simulink model "Cmd_HacheurF"  (R2016a)
settings: Solver=ode1  StartTime=0.0  StopTime=0.05  FixedStep=Te  RelTol=1e-3
values from neighbouring files (symbols this model uses):
  A = [-R/L -1/L;1/Cdc -1/(Cdc*Rch)]    [Param.m]
  Ad = [1-Te*R/L -Te/L;Te/Cdc 1-Te/(Cdc*Rch)]    [Param.m]
  B = [1/L;0]    [Param.m]
  Bd = [Te/L;0]    [Param.m]
  C = [0 1]    [Param.m]
  Cd = [0 1]    [Param.m]
  Cdc = 200e-6    (= 0.0002)    [Param.m]
  K = place(A,B,[p1BF;p2BF])    [Param.m]
  L = 12.5e-3    (= 0.0125)    [Param.m]
  LOBS = LOBS_T'    [Param.m]
  LOBSd = Te*LOBS    [Param.m]
  N = inv(-C*inv(A-B*K)*B)    [Param.m]
  R = 0.3    [Param.m]
  Rch = 50    [Param.m]
  Te = 20e-6    (= 2e-05)    [Param.m]
  X_0 = [0;0]    [Param.m]
settings Model: Creator=Wissem  LastModifiedBy=dell

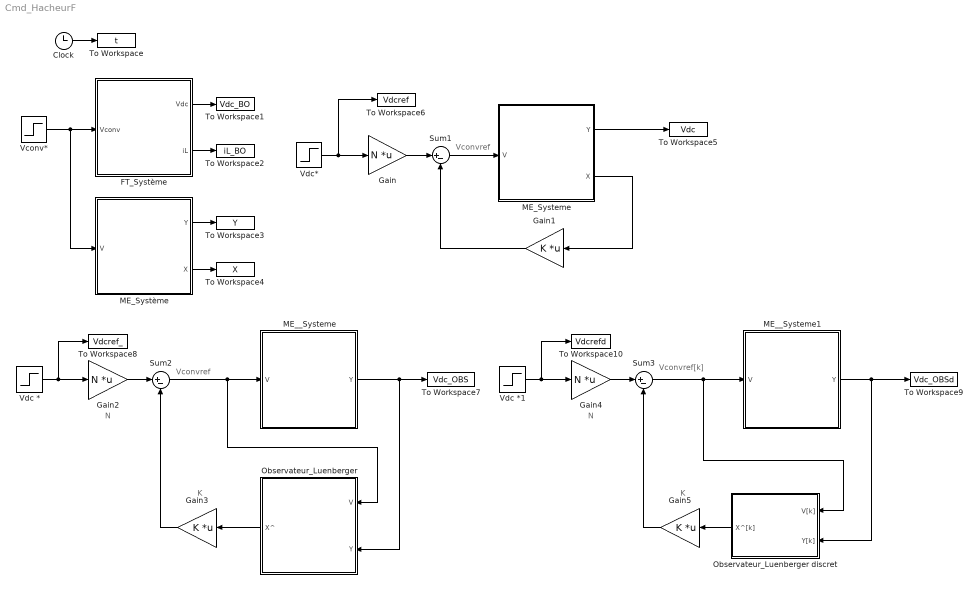
== system Cmd_HacheurF ==
  note: N
  note: K
  note: Vconvref
  note: Vconvref
  note: N
  note: K
  note: Vconvref[k]
  Clock : Clock
  FT_Système : Subsystem
  Gain : Gain  Gain=N  Multiplication=Matrix(K*u)
  Gain1 : Gain  Gain=K  Multiplication=Matrix(K*u) (u vector)
  Gain2 : Gain  Gain=N  Multiplication=Matrix(K*u)
  Gain3 : Gain  Gain=K  Multiplication=Matrix(K*u) (u vector)
  Gain4 : Gain  Gain=N  Multiplication=Matrix(K*u)
  Gain5 : Gain  Gain=K  Multiplication=Matrix(K*u) (u vector)
  ME_Systeme : Subsystem
  ME_Système : Subsystem
  ME__Systeme : Subsystem
  ME__Systeme1 : Subsystem
  Observateur_Luenberger : Subsystem
  Observateur_Luenberger discret : Subsystem
  Sum1 : Sum  Inputs=|+-
  Sum2 : Sum  Inputs=|+-
  Sum3 : Sum  Inputs=|+-
  To Workspace : ToWorkspace  VariableName=t  SampleTime=-1
  To Workspace1 : ToWorkspace  VariableName=Vdc_BO  SampleTime=-1
  To Workspace10 : ToWorkspace  VariableName=Vdcrefd  SampleTime=-1
  To Workspace2 : ToWorkspace  VariableName=iL_BO  SampleTime=-1
  To Workspace3 : ToWorkspace  VariableName=Y  SampleTime=-1
  To Workspace4 : ToWorkspace  VariableName=X  SampleTime=-1
  To Workspace5 : ToWorkspace  VariableName=Vdc  SampleTime=-1
  To Workspace6 : ToWorkspace  VariableName=Vdcref  SampleTime=-1
  To Workspace7 : ToWorkspace  VariableName=Vdc_OBS  SampleTime=-1
  To Workspace8 : ToWorkspace  VariableName=Vdcref_  SampleTime=-1
  To Workspace9 : ToWorkspace  VariableName=Vdc_OBSd  SampleTime=-1
  Vconv* : Step  Time=0  After=100  SampleTime=0
  Vdc * : Step  Time=0  After=100  SampleTime=0
  Vdc *1 : Step  Time=0  After=100  SampleTime=0
  Vdc* : Step  Time=0  After=100  SampleTime=0
  wires:
  Vconv*/1 -> ME_Système/1(V), FT_Système/1(Vconv)
  Clock/1 -> To Workspace/1
  FT_Système/1(Vdc) -> To Workspace1/1
  FT_Système/2(iL) -> To Workspace2/1
  ME_Système/1(Y) -> To Workspace3/1
  ME_Système/2(X) -> To Workspace4/1
  Gain1/1 -> Sum1/2
  Gain/1 -> Sum1/1
  Vdc*/1 -> To Workspace6/1, Gain/1
  Sum1/1 -> ME_Systeme/1(V)
  ME_Systeme/1(Y) -> To Workspace5/1
  ME_Systeme/2(X) -> Gain1/1
  Gain3/1 -> Sum2/2
  Gain2/1 -> Sum2/1
  Vdc */1 -> Gain2/1, To Workspace8/1
  Sum2/1 -> Observateur_Luenberger/1(V), ME__Systeme/1(V)
  ME__Systeme/1(Y) -> Observateur_Luenberger/2(Y), To Workspace7/1
  Observateur_Luenberger/1(X^) -> Gain3/1
  Gain5/1 -> Sum3/2
  Gain4/1 -> Sum3/1
  Vdc *1/1 -> To Workspace10/1, Gain4/1
  Sum3/1 -> Observateur_Luenberger discret/1(V[k]), ME__Systeme1/1(V)
  ME__Systeme1/1(Y) -> Observateur_Luenberger discret/2(Y[k]), To Workspace9/1
  Observateur_Luenberger discret/1(X^[k]) -> Gain5/1

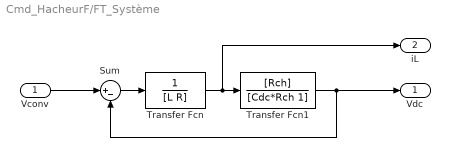
== system Cmd_HacheurF/FT_Système ==
  Vconv : Inport
  Sum : Sum  Inputs=|+-
  Transfer Fcn : TransferFcn  Denominator=[L R]
  Transfer Fcn1 : TransferFcn  Numerator=[Rch]  Denominator=[Cdc*Rch 1]
  Vdc : Outport
  iL : Outport  Port=2
  wires:
  Transfer Fcn/1 -> iL/1, Transfer Fcn1/1
  Transfer Fcn1/1 -> Vdc/1, Sum/2
  Sum/1 -> Transfer Fcn/1
  Vconv/1 -> Sum/1

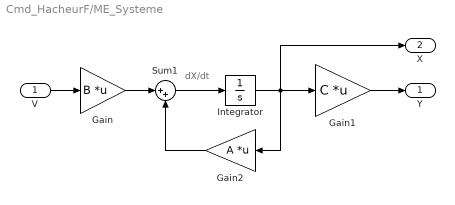
== system Cmd_HacheurF/ME_Systeme ==
  note: dX/dt
  V : Inport
  Gain : Gain  Gain=B  Multiplication=Matrix(K*u)
  Gain1 : Gain  Gain=C  Multiplication=Matrix(K*u) (u vector)
  Gain2 : Gain  Gain=A  Multiplication=Matrix(K*u) (u vector)
  Integrator : Integrator  InitialCondition=X_0
  Sum1 : Sum  Inputs=|++
  Y : Outport
  X : Outport  Port=2
  wires:
  Gain2/1 -> Sum1/2
  Integrator/1 -> Gain1/1, X/1, Gain2/1
  Gain1/1 -> Y/1
  Sum1/1 -> Integrator/1
  Gain/1 -> Sum1/1
  V/1 -> Gain/1

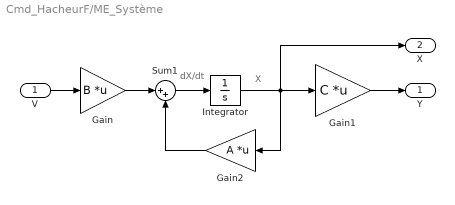
== system Cmd_HacheurF/ME_Système ==
  note: X
  note: dX/dt
  V : Inport
  Gain : Gain  Gain=B  Multiplication=Matrix(K*u)
  Gain1 : Gain  Gain=C  Multiplication=Matrix(K*u) (u vector)
  Gain2 : Gain  Gain=A  Multiplication=Matrix(K*u) (u vector)
  Integrator : Integrator  InitialCondition=X_0
  Sum1 : Sum  Inputs=|++
  Y : Outport
  X : Outport  Port=2
  wires:
  V/1 -> Gain/1
  Gain/1 -> Sum1/1
  Sum1/1 -> Integrator/1
  Gain1/1 -> Y/1
  Integrator/1 -> Gain2/1, X/1, Gain1/1
  Gain2/1 -> Sum1/2

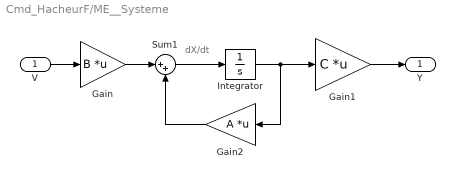
== system Cmd_HacheurF/ME__Systeme ==
  note: dX/dt
  V : Inport
  Gain : Gain  Gain=B  Multiplication=Matrix(K*u)
  Gain1 : Gain  Gain=C  Multiplication=Matrix(K*u) (u vector)
  Gain2 : Gain  Gain=A  Multiplication=Matrix(K*u) (u vector)
  Integrator : Integrator  InitialCondition=X_0
  Sum1 : Sum  Inputs=|++
  Y : Outport
  wires:
  V/1 -> Gain/1
  Gain/1 -> Sum1/1
  Sum1/1 -> Integrator/1
  Gain1/1 -> Y/1
  Integrator/1 -> Gain2/1, Gain1/1
  Gain2/1 -> Sum1/2

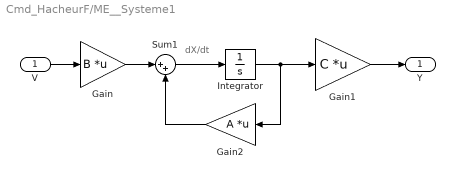
== system Cmd_HacheurF/ME__Systeme1 ==
  note: dX/dt
  V : Inport
  Gain : Gain  Gain=B  Multiplication=Matrix(K*u)
  Gain1 : Gain  Gain=C  Multiplication=Matrix(K*u) (u vector)
  Gain2 : Gain  Gain=A  Multiplication=Matrix(K*u) (u vector)
  Integrator : Integrator  InitialCondition=X_0
  Sum1 : Sum  Inputs=|++
  Y : Outport
  wires:
  Gain2/1 -> Sum1/2
  Integrator/1 -> Gain1/1, Gain2/1
  Gain1/1 -> Y/1
  Sum1/1 -> Integrator/1
  Gain/1 -> Sum1/1
  V/1 -> Gain/1

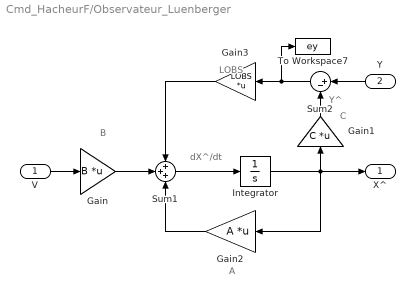
== system Cmd_HacheurF/Observateur_Luenberger ==
  note: Y^
  note: C
  note: LOBS
  note: A
  note: B
  note: dX^/dt
  V : Inport
  Y : Inport  Port=2
  Gain : Gain  Gain=B  Multiplication=Matrix(K*u)
  Gain1 : Gain  Gain=C  Multiplication=Matrix(K*u) (u vector)
  Gain2 : Gain  Gain=A  Multiplication=Matrix(K*u) (u vector)
  Gain3 : Gain  Gain=LOBS  Multiplication=Matrix(K*u) (u vector)
  Integrator : Integrator  InitialCondition=[0;0]
  Sum1 : Sum  Inputs=+++
  Sum2 : Sum  Inputs=|+-
  To Workspace7 : ToWorkspace  VariableName=ey  SampleTime=-1
  X^ : Outport
  wires:
  Integrator/1 -> X^/1, Gain1/1, Gain2/1
  Sum1/1 -> Integrator/1
  V/1 -> Gain/1
  Y/1 -> Sum2/1
  Sum2/1 -> To Workspace7/1, Gain3/1
  Gain/1 -> Sum1/2
  Gain2/1 -> Sum1/3
  Gain3/1 -> Sum1/1
  Gain1/1 -> Sum2/2

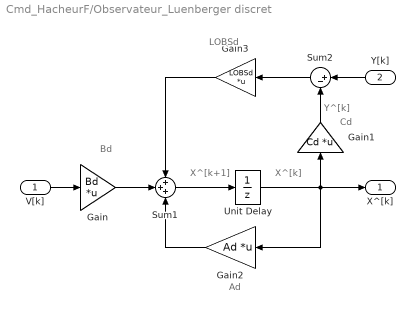
== system Cmd_HacheurF/Observateur_Luenberger discret ==
  note: X^[k+1]
  note: Bd
  note: Ad
  note: LOBSd
  note: Cd
  note: Y^[k]
  note: X^[k]
  V[k] : Inport
  Y[k] : Inport  Port=2
  Gain : Gain  Gain=Bd  Multiplication=Matrix(K*u)
  Gain1 : Gain  Gain=Cd  Multiplication=Matrix(K*u) (u vector)
  Gain2 : Gain  Gain=Ad  Multiplication=Matrix(K*u) (u vector)
  Gain3 : Gain  Gain=LOBSd  Multiplication=Matrix(K*u) (u vector)
  Sum1 : Sum  Inputs=+++
  Sum2 : Sum  Inputs=|+-
  Unit Delay : UnitDelay  SampleTime=Te
  X^[k] : Outport
  wires:
  Gain1/1 -> Sum2/2
  Gain3/1 -> Sum1/1
  Gain2/1 -> Sum1/3
  Gain/1 -> Sum1/2
  Sum2/1 -> Gain3/1
  Y[k]/1 -> Sum2/1
  V[k]/1 -> Gain/1
  Sum1/1 -> Unit Delay/1
  Unit Delay/1 -> Gain2/1, Gain1/1, X^[k]/1
